simulink model "ADC_RoadRunner"  (R2024b)
settings: Solver=ode23tb  StartTime=0  StopTime=20  FixedStep=0.01  RelTol=1e-3
model workspace (MAT data in the model file):
  finalint = 0
  firstWarning = 1
  originalScenarioChecksum = '114339432DE22364D47BB28FC96DC10C'
undefined symbols (not defined in the file): curvature, DefaultGear, Defined, DEND_B, DEND_S, DEND_T, direction, DiscIntNeverNeededParam, driving, dspblkCoreblockFVToolHelper, Ego, fractalcoef, gcbh, gradbp, L, Lane, LF, LR, m, MAX_BRAKE, MAX_STEER, MAX_TORQUE, maxNumActors, MCAR, MIN_BRAKE, MIN_STEER, MIN_TORQUE, n, NUMD_B, NUMD_S, NUMD_T, Pose, psi_o, R, RRdamp, sigbuilder_block, STEER_RATIO, Tdead, thetaRefs, TrackWidth, ts, Ts, User, Vdead, Velocity, WB, xRef2s, yRef2s
libraries: simulink x9, roadrunnerscenario x7, simulink_extras x4, drivingscenarioandsensors x3, sensorinslib x2, robotalgslib x1, mpcadaslib x1, drivingvehiclecontroller x1, slpidlib x1, sensorgpslib x1, mspsensorlib x1, LaneDetection x1
(part 4 of 4)

== matlab function ADC_RoadRunner/Subsystem1/MATLAB Function ==
  data: ttc output; dist output; left output; right output; LL_avail output; RL_avail output; tend2stay output; ego input; act input; LaneBounds input; RoadSpeed input; ego_vel output; stay output; LL_Change output; RL_Change output; y_lane output; LCinProgress input
function [ttc,dist,left,right,LL_avail,RL_avail,tend2stay,ego_vel,stay,LL_Change,RL_Change,y_lane] = fcn(ego,act,LaneBounds,RoadSpeed, LCinProgress)                       


%% Major tasks to look into

% Check the performance while transitioning into another lane 
% Lane change output when the ego on extreme lanes.
% Develop code to handle lane changes on road curvatures
% Integrate with the trajectory generation and check the perfomance
% Convert the code to ego vehicle coordinates


%%
%define some parameters
r_c = 20; %range considered to MIOs
t_min =  2;

num_actors = length(act.Actors);
%num_lanes = length(LaneBounds.LaneBoundaries)-1;


%% Using sensor data 
% TracksNum = Tracking.NumTracks;
% 
% 
% for t = 1:TracksNum
%     ObjectID(t) = Tracking.Tracks(t).ObjectClassID;
%     TrackPos(:,t) = Tracking.Tracks(t).State(1:2:5);
%     TrackVel(:,t) = Tracking.Tracks(t).State(2:2:6);

%% ego position and  velocity magnitude
ego_pos = ego.Position;
ego_vel = ego.Velocity(1);  % velocity

%ttc: (array) : agent.relative position / abs(relative velocity)
ttc = zeros(1,num_actors);
left = zeros(1,num_actors);
right = zeros(1,num_actors);

dist =  zeros(1,num_actors);
tend2stay=1;

%%
y_lane = zeros(1,length(LaneBounds.LaneBoundaries))

for l=1:length(y_lane)
    y_lane(l)=LaneBounds.LaneBoundaries(l).Coordinates(end,2)
end

%%
for i= 1:num_actors

    % Grab actor positions and velocities
    actor_pos = act.Actors(i).Position;   
    actor_vel = act.Actors(i).Velocity(1);  % x-component velocity

    %relative velocity of the agent
    rel_vel = actor_vel - ego_vel;


    %% Check if the actor is within a r_c range. If it is out of range, pass lane change as '1' automatically.

   dist(i) = norm([actor_pos(1) actor_pos(2)]-[ego_pos(1) ego_pos(2)]);
        
    if dist(i) > r_c
        left(i)=1;
        right(i)=1;
        continue
    end

    %% Check if the actor is in the same lane as that of ego

    % If the actor and ego are in the same lane, it is considered a lead/following vehicle in the same lane and by defualt, the lane change flag is 1.

    if (actor_pos(2)< (ego_pos(2)+0.5) && actor_pos(2) > (ego_pos(2)-0.5))
        if (rel_vel < 0 && ego_vel < (RoadSpeed+5) && actor_pos(1) > ego_pos(1) )
            left(i) =1;
            right(i)=1;
            tend2stay=0;        % we need to incorporate too slow condition even when the relative velocity is greater than 0.

        elseif (rel_vel < 0 && ego_vel < (RoadSpeed+5) && actor_pos(1) < ego_pos(1) )
            left(i) =1;
            right(i)=1;
            tend2stay=1;
        end

        continue
    end

    
    %% calculate ttc for the rest of the vehicles


    ttc(i) = (actor_pos(1)-ego_pos(1))/abs(rel_vel);

    % checking conditions for other surrounding actors

    % all actors on the left lane of the ego vehicle
%%
    if actor_pos(2)-ego_pos(2) > 0  

        if and(rel_vel>0, ttc(i) > t_min)  % target vehicles on the front of ego vehicle (any lane)
    
            left(i)=1; 
            right(i)=1;
    
        elseif (ttc(i)<0 && rel_vel<0 && abs(ttc(i)) > t_min)    % target vehicle on the back of ego vehicle (ttc<0) (any lane)
            left(i) =1;
            right(i)=1;
    
        else 
            left(i) =0;
            right(i)=1;
    
        end

    % all actors on the right lane of the ego vehicle

    elseif actor_pos(2)-ego_pos(2) < 0
         
        if and(rel_vel>0, ttc(i) > t_min)  % target vehicles on the front of ego vehicle (any lane)
    
            left(i)=1;
            right(i)=1;
    
        elseif (ttc(i)<0 && rel_vel<0 && abs(ttc(i)) > t_min)    % target vehicle on the back of ego vehicle (ttc<0) (any lane)
            left(i) =1;
            right(i)=1;
    
        else 
            left(i) =1;
            right(i)=0;
    
        end
    end
%%

end

%% check if the vehicle is in the extreme end lanes

    if ego_pos(2)<y_lane(1) && ego_pos(2)>y_lane(2)

        LL=0; RL=1;
    elseif ego_pos(2) > y_lane(end) && ego_pos(2) < y_lane(end-1)
        RL=0; LL=1;
    else 

        RL=1;LL=1;
    end

%%
LL_avail = all(left) %&& LL;

RL_avail = all(right) %&& RL               %&& ~lcLeft ; this can be decided later 


%% final commands

stay = tend2stay || ~(tend2stay || LL_avail || RL_avail);
LL_Change =  ~tend2stay && LL_avail ;

RL_Change =  ~tend2stay && RL_avail && ~LL_Change ;
LCFlag = ~stay;
if LCFlag && LCinProgress
    LCFlag = false;
    stay = ~LCFlag;
end

%% 






end

== matlab function ADC_RoadRunner/Environment & Data/MATLAB Function ==
  data: states input; stateDynamics output; inputCmd input
function stateDynamics  = StateEstimator(states, inputCmd)


    % Model Parameters:
    J = 4000; 
    yawPolarIzz = 2050; %
    vehicleMass = 2000;
    lFront = 1.3425;
    lRear = 1.3425;
    corneringStiffnessFront = 12e3*100; 
    corneringStiffnessRear = 12e3*100;

    % Inputs
    accel = inputCmd(1);
    steerDelta = inputCmd(2);

    % States
    x = states(1);
    y = states(2);
    vx = states(3);
    vy = states(4);
    w = states(5);
    psi = states(6);
    
    

    alphaFront = atan2(vy + lFront*w)/vx - steerDelta;
    alphaRear = (vy - lRear*w)/vx;

    % Model - Dynamics Equations:
    stateDynamics = zeros(6,1);
    xDot = vx*cos(psi) - vy*sin(psi);
    yDot = vx*sin(psi)) + vy*cos(psi);

    vxDot = vy*w + 1/m();
    vyDot = ;
    psiDot = w;
    wDot = ;

    stateDynamics = [xDot; yDot; vxDot; vyDot; psiDot; wDot];

end

== stateflow chart ADC_RoadRunner/Vehicle Dynamics/Vehicle Dynamics/Engineer Steer Brake Dynamics/GearSelection1 ==
  state Park
    CurrGear = 0;
  state Reverse
    CurrGear = -1;
  state drive
    CurrGear = 1;
  (default) -> (junction 12)
  (junction 12) -> Reverse [order 3] : [DefaultGear == -1]
  (junction 12) -> drive [order 2] : [DefaultGear == 1]
  (junction 12) -> Park [order 1] : [DefaultGear == 0]
  (junction 12) -> Park [order 4] : %fallback to park
  drive -> Park [order 2] : [gear_cmd == 0 && allowShift(vc,Tbrake)]
  Park -> Reverse [order 2] : [gear_cmd == -1 && allowShift(vc,Tbrake)]
  Park -> drive [order 1] : [gear_cmd == 1 && allowShift(vc,Tbrake)]
  Reverse -> Park [order 2] : [gear_cmd == 0 && allowShift(vc,Tbrake)]
  drive -> Reverse [order 1] : [gear_cmd == -1 && allowShift(vc,Tbrake)]
  Reverse -> drive [order 1] : [gear_cmd == 1 && allowShift(vc,Tbrake)]
  data: Tdead parameter; Vdead parameter; vel function_input; brakeT function_input; allow function_output; CurrGear output; Tbrake input; vc input; gear_cmd input; DefaultGear parameter
  function allow = allowShift(vel, brakeT):
    | function allow = allowShift(vel, brakeT)
    | allow = (abs(vel) <= Vdead) && (abs(brakeT)>Tdead);
    | end

== matlab function ADC_RoadRunner/Vehicle Dynamics/Vehicle Dynamics/Engineer Steer Brake Dynamics/Compute Net Torque ==
  data: gear input; Tnet output; Tengine input; Tbrake input; vc input
function Tnet  = net_torque(gear,Tengine,Tbrake,vc)

%  --set engine torque based on current gear selection

if (gear == 0)
    %  --vehicle is in PARK, so force engine torque to zero
    Tengine = 0;
end

Tnet = Tengine + Tbrake*tanh(5*vc);

end

== matlab function ADC_RoadRunner/Vehicle Dynamics/Vehicle Dynamics/Engineer Steer Brake Dynamics/gear selection state machine ==
  data: gear output; gear_cmd input; vc input; Tbrake input; Tdead input; Vdead input
function gear = gear_change_FSM(gear_cmd,vc,Tbrake,Tdead,Vdead)

persistent GEAR

%  The vehicle gear can take on one of the following enumerated values:
%  -1 = REVERSE
%   0 = PARK
%   1 = DRIVE

%  --initialize the local persistent variables

if isempty(GEAR)
    %  --default gear at startup is PARK
    %  Note:  Change this to 1 if you want car to initialize in DRIVE
    GEAR = 0;
end


%  --evaluate the gear change finite state machine

switch GEAR
    case 0  % vehicle is in PARK
        if (gear_cmd == 1)
            %  --check to see if we can shift to DRIVE
            if ((abs(vc) <= Vdead) && (abs(Tbrake) > Tdead))
                %  --shift to DRIVE
                GEAR = 1;
            end
            
        elseif (gear_cmd == 2)
            %  --check to see if we can shift to REVERSE
            if ((abs(vc) <= Vdead) && (abs(Tbrake) > Tdead))
                %  --shift to REVERSE
                GEAR = 2;
            end
        end
        
    case 1  % vehicle is in DRIVE
        if (gear_cmd == 0)
            %  --check to see if we can shift to PARK
            if ((abs(vc) <= Vdead) && (abs(Tbrake) > Tdead))
                %  --shift to PARK
                GEAR = 0;
            end
            
        elseif (gear_cmd == 2)
            %  --check to see if we can shift to REVERSE
            if ((abs(vc) <= Vdead) && (abs(Tbrake) > Tdead))
                %  --shift to REVERSE
                GEAR = 2;
            end
        end
        
    case -1  % vehicle is in REVERSE
        if (gear_cmd == 0)
            %  --check to see if we can shift to PARK
            if ((abs(vc) <= Vdead) && (abs(Tbrake) > Tdead))
                %  --shift to PARK
                GEAR = 0;
            end
            
        elseif (gear_cmd == 1)
            %  --check to see if we can shift to DRIVE
            if ((abs(vc) <= Vdead) && (abs(Tbrake) > Tdead))
                %  --shift to DRIVE
                GEAR = 1;
            end
        end
        
    otherwise  %  --should never be here
        if (vc > Vdead)
            %  --moving forward, so must be in DRIVE
            GEAR = 1;
        elseif (vc < -Vdead)
            %  --moving backward, so must be in REVERSE
            GEAR = 2;
        else
            %  --vehicle stoppped, so must be in PARK
            GEAR = 0;
        end

end


%  --output the current actual gear setting

gear = GEAR;

return

== matlab function ADC_RoadRunner/Behavioural Planner/MATLAB Function3 ==
  data: Dest input; D2D output; CurrentPose input
function D2D = fcn(Dest, CurrentPose)
%CurrentPose(2) = -CurrentPose(2);
%D2D = norm(Dest - CurrentPose(1:2)');
Dest = [Dest(2) Dest(1)]; 
CurrentPose = [CurrentPose(2) CurrentPose(1)];
D2D = norm(Dest - CurrentPose(1:2));
% D2D=sqrt((CurrentPose(1)-Dest(1,1))^2+(CurrentPose(2)-Dest(1,2))^2);
end

== stateflow chart ADC_RoadRunner/Behavioural Planner/Chart ==
  settings: updateMethod=DISCRETE  sampleTime=Ts
  state Stationary
    en,du:
    VelCmd = 0;
    CurrentVelCmd = VelCmd;
    Navi = 0;
    Trans = 0;
    StopSim = 0;
    Tgap = 1;
    HoldBrake = 1;
    Braking = 0;
    SpeedUp = 0;
  state Navigation
    state RailCrossing [commented out]
      state Stop [commented out]
        en:
        VelCmd = 0;
        Braking = 1;
        CurrentVelCmd = VelCmd;
      state Approaching [commented out]
        en:
        Braking = 1;
        Tgap = 0;
        Trans = 0;
      state Transition [commented out]
        en:
        Tgap = 1;
        Trans = 1;
        Braking = 0;
        VelCmd = SceneSpeed;
        CurrentVelCmd = VelCmd;
      state ExitScene [commented out]
        en:
        ExitFlag = 1;
      (default) -> Navigation.RailCrossing.Approaching [commented out]
      Navigation.RailCrossing.Approaching -> Navigation.RailCrossing.Stop [commented out] : [D2S <= 6 && (RRCross == 1 || ObjectDist <= TransDist)]
      Navigation.RailCrossing.Transition -> Navigation.RailCrossing.Approaching [commented out] : [ObjectDist <= TransDist]
      Navigation.RailCrossing.Approaching -> Navigation.RailCrossing.Transition [commented out] : [RRCross == 0 && ObjectDist > TransDist && D2S <= 6]
      Navigation.RailCrossing.Stop -> Navigation.RailCrossing.Transition [commented out] : [RRCross == 0 && ObjectDist > TransDist]
      Navigation.RailCrossing.Approaching -> Navigation.RailCrossing.ExitScene [commented out] : [SceneID ~= 10]
      Navigation.RailCrossing.Transition -> Navigation.RailCrossing.ExitScene [commented out] : [SceneID == 0]
    state RoundAbout
      state Approaching
        en:
        Braking = 1;
        Trans = 0;
        Tgap = 0;
      state Stop
        en:
        VelCmd = 0;
        Braking = 1;
        CurrentVelCmd = VelCmd;
      state ExitScene
        en:
        ExitFlag = 1;
      state Transition
        en:
        Tgap = 1;
        Trans = 1;
        Braking = 0;
        VelCmd = SceneSpeed;
        CurrentVelCmd = VelCmd;
      (default) -> Navigation.RoundAbout.Approaching
      Navigation.RoundAbout.Approaching -> Navigation.RoundAbout.Stop [order 1] : [D2S <= 6]
      Navigation.RoundAbout.Stop -> Navigation.RoundAbout.Transition : [Clear2Go == 1]
      Navigation.RoundAbout.Approaching -> Navigation.RoundAbout.ExitScene [order 2] : [SceneID ~= 9]
      Navigation.RoundAbout.Transition -> Navigation.RoundAbout.ExitScene : [SceneID == 0]
    state DestCheck
      en,du:
      % dest reached?
      (default) -> (junction 47)
      (junction 47) -> (junction 48) [order 1] : [D2D < 2]
      (junction 47) -> (junction 49) [order 2] : {DestReached = 0;}
      (junction 48) -> (junction 50) : {DestReached = 1;}
      (junction 50) -> (junction 49) : {StopSim = 1;}
      (junction 49) -> (junction 51)
    state TrafficLight [commented out]
      note: Yellow light duration is 1s
      state Stop [commented out]
        en:
        Braking = 1;
        VelCmd = 0;
        CurrentVelCmd = VelCmd;
      state Approaching [commented out]
        en:
        Tgap = 0;
        Trans = 0;
        T2S = 0;
        %if TLstate(1,4) == 1
        Braking = 1;
        %else
        % ACC = 0;
        %end
      state DecisionOnYellow [commented out]
        en:
        T2S = D2S/EgoSpeed;
      state Transition [commented out]
        en:
        Trans = 1;
        Braking = 0;
        Tgap = 1;
        VelCmd = SceneSpeed;
        CurrentVelCmd = VelCmd;
      state ExitScene [commented out]
        en:
        ExitFlag = 1;
      DecisionOnYellow -> Navigation.TrafficLight.Approaching [commented out] : [T2S > 1.2]
      (default) -> Navigation.TrafficLight.Approaching [commented out]
      Navigation.TrafficLight.Approaching -> Navigation.TrafficLight.Stop [commented out] : [D2S <= 6]
      Navigation.TrafficLight.Stop -> Navigation.TrafficLight.Transition [commented out] : [TLstate(1,4) == 3 && ObjectDist > TransDist]
      Navigation.TrafficLight.Transition -> Navigation.TrafficLight.Approaching [commented out] : [TLstate(1,4) == 1  || ObjectDist < TransDist]
      Navigation.TrafficLight.Approaching -> Navigation.TrafficLight.Transition [commented out] : [TLstate(1,4) == 3 && ObjectDist > TransDist]
      Navigation.TrafficLight.Approaching -> Navigation.TrafficLight.ExitScene [commented out] : [SceneID ~= 8]
      Navigation.TrafficLight.Transition -> DecisionOnYellow [commented out] : [TLstate(1,4) == 2]
      DecisionOnYellow -> Navigation.TrafficLight.Transition [commented out] : [T2S <= 1.2]
      Navigation.TrafficLight.Transition -> Navigation.TrafficLight.ExitScene [commented out] : [SceneID == 0]
    state Drive
      en :
      HoldBrake = 0;
      SpeedUp = 1;
      VelCmd = RoadSpeed;
      CurrentVelCmd = VelCmd;
      ExitFlag = 0;
    state Go
      en:
      %VelCmd = RoadSpeed;
      %CurrentVelCmd = VelCmd;
      Trans = 0;
      ExitFlag = 0;
      Braking = 0;
      HoldBrake = 0;
      SpeedUp = 0;
    state StopSign
      state StoptSign4way
        state CheckInt
          du:
          % stopped?
          % ss priority?
        state CheckSS
          % stopped?
          % ss priority?
        state Transition
          en:
          % stay here while trans?!
          % while ~crossedLimitLine of TargetLane
          Trans = 1;
          Braking = 0;
          Tgap = 1;
          VelCmd = SceneSpeed;
          CurrentVelCmd = VelCmd;
        state ExitScene
          en:
          ExitFlag = 1;
        (default) -> Navigation.StopSign.StoptSign4way.CheckSS
        Navigation.StopSign.StoptSign4way.CheckSS -> Navigation.StopSign.StoptSign4way.CheckInt : [EgoSpeed < VelStop]
        Navigation.StopSign.StoptSign4way.CheckInt -> Navigation.StopSign.StoptSign4way.Transition : [egoSSPriority == 1 && Clear2Go == 1]
        Navigation.StopSign.StoptSign4way.Transition -> Navigation.StopSign.StoptSign4way.ExitScene : [SceneID == 0 && after(2,sec)]
      state SStype
        state Stop
          en:
          %VelCmd = 0;
          Braking = 1;
          SpeedUp = 0;
          CurrentVelCmd = VelCmd;
        state Approaching
          en:
          %VelCmd = ApproachingSpeed;
          % Braking = 1;
          Trans = 0;
          Tgap = 0;
        Navigation.StopSign.SStype.Stop -> 410 [order 1] : [numSS == 4]
        (default) -> Navigation.StopSign.SStype.Approaching
        Navigation.StopSign.SStype.Approaching -> Navigation.StopSign.SStype.Stop : [D2S <= 25]
        Navigation.StopSign.SStype.Stop -> 414 [order 2] : [numSS == 2]
      state StopSign2way
        state CheckInt
          en:
          %VelCmd = 0;
          HoldBrake = 1;
          CurrentVelCmd = VelCmd;
        state CheckSS
          % stopped?
          % ss priority?
        state Transition1
          en:
          % stay here while trans?!
          % while ~crossedLimitLine of TargetLane
          Trans = 1;
          Braking = 0;
          HoldBrake = 0;
          SpeedUp = 1;
          Tgap = 1;
          VelCmd = SceneSpeed;
          CurrentVelCmd = VelCmd;
        state ExitScene1
          en:
          ExitFlag = 1;
        (default) -> Navigation.StopSign.StopSign2way.CheckSS
        Navigation.StopSign.StopSign2way.CheckSS -> Navigation.StopSign.StopSign2way.CheckInt : [EgoSpeed < VelStop]
        Navigation.StopSign.StopSign2way.CheckInt -> Transition1 : [egoSSPriority == 1 && after(3,sec) && ToAClearance == 1]
        Transition1 -> Navigation.StopSign.StopSign2way.CheckInt [order 2] : [ToAClearance == 0]
        Transition1 -> ExitScene1 [order 1] : [SceneID == 0 && after(3,sec) && egoExit == 1]
      (default) -> SStype
      416 -> StoptSign4way
      411 -> StopSign2way
    Go -> RailCrossing [commented out] : [SceneID == 10]
    Drive -> RailCrossing [commented out] : [SceneID == 10]
    RailCrossing -> Go [commented out] : [ExitFlag == 1]
    Go -> RoundAbout [order 2] : [SceneID == 9]
    Drive -> RoundAbout [order 1] : [SceneID == 9]
    RoundAbout -> Go : [ExitFlag == 1]
    (default) -> DestCheck
    Drive -> TrafficLight [commented out] : [SceneID == 8]
    DestCheck -> Drive : [DestReached == 0]
    Go -> TrafficLight [commented out] : [SceneID == 8]
    Drive -> DestCheck [order 3] : [D2D < 2]
    TrafficLight -> Go [commented out] : [ExitFlag == 1]
    Drive -> StopSign [order 2] : [SceneID == 7]
    StopSign -> Go : [ExitFlag == 1]
    Go -> DestCheck [order 1] : [SceneID == 0]
    Go -> StopSign [order 3] : [SceneID == 7]
  (default) -> Stationary
  Stationary -> Navigation : [Navigate == 1]
  Navigation -> Stationary : [Navigate == 0 || DestReached == 1]
  data: TLstate input; numSS input; egoExit input; ToAClearance input; TransDist input; ApproachingSpeed input; EgoSpeed input; ObjectDist input; SceneSpeed input; SDist input; RRCross input; D2S input; DestReached local; Navigate input; ExitFlag local; D2D input; Clear2Go input; RoadSpeed input; CurrentVelCmd local; Navi local; VelCmd output; HoldBrake output; SceneID input; Tgap output; Trans output; StopSim output; Braking output; T2S local; VelStop input; egoSSPriority input; SpeedUp output

== matlab function ADC_RoadRunner/Behavioural Planner/MATLAB Function ==
  data: u input; y output
function y = fcn(u)

y = u;

== matlab function ADC_RoadRunner/Subsystem1/Subsystem/Function-Call Subsystem/MATLAB Function1 ==
  data: EgoPosition input; MIOPos input; curvature input; MIOVel input; V_i input; xd output; yd output; laneL input; laneR input; V_desired input; LCinProgress output
function [xd,yd,LCinProgress] = traj(EgoPosition,MIOPos,curvature,MIOVel, V_i, laneL, laneR, V_desired)
Vx_i =0;Vx_f=0;Vy_i=0;Vy_f=0;Ax_i=0;Ax_f=0;Ay_i=0;Ay_f=0;T_i=0;T_f=0;V_f=0;A_f=0;x_set=0;y_set=0;theta4=0;

P = zeros(6,6);
% xq = zeros(1,size(RefPath,1)); yq = zeros(1,size(RefPath,2));
EgoPosition(1,2)=-EgoPosition(1,2);
x_init= EgoPosition(1,1)+2; y_init = EgoPosition(1,2)-2;
% xq = RefPath(:,1)'; 
% yq = RefPath(:,2)';
num_foc_t = 98;
V_max= V_desired; ad_n=0; vd_n=MIOVel; wd_n=vd_n*curvature;
lane_width = 3.6 * (laneL-laneR); % +1 if left of current lane and -1 if right of current lane(rahul flipped)
xd = zeros(num_foc_t+1,1); 
yd = zeros(num_foc_t+1,1);
xf =0; 
yf = 0;

    %xf = [EgoPosition(1,1)+ MIOPos(1) ]; yf = [ EgoPosition(1,2)+ MIOPos(2) + lane_width];  
    xf = [EgoPosition(1,1)+ 20 ]; yf = [EgoPosition(1,2)+ lane_width]; % 80
    V_f = V_max;
    W_f = V_f*curvature;
    A_f = 0;

    %dist2crash = sqrt((x_init-MIOPos(1))^2+(y_init-MIOPos(2))^2);
    %dist2crash = 40;
    %T_f = abs(dist2crash/(MIOVel-V_i));
    T_f = 3;
    P = [1, T_i, T_i^2, T_i^3, T_i^4, T_i^5;
         0, 1, 2*T_i, 3*T_i^2, 4*T_i^3, 5*T_i^4;
         0, 0, 2, 6*T_i, 12*T_i^2, 20*T_i^3;
         1, T_f, T_f^2, T_f^3, T_f^4, T_f^5;
         0, 1, 2*T_f, 3*T_f^2, 4*T_f^3, 5*T_f^4;
         0, 0, 2, 6*T_f, 12*T_f^2, 20*T_f^3];

%     mtang4 = (yq(1,index+2)-yq(1,index+1))/(xq(1,index+2)-xq(1,index+1));

    Vx_i = vd_n*cos(theta4); 
    Vy_i = vd_n*sin(theta4); 
    Ax_i = ad_n*cos(theta4)-vd_n*sin(theta4)*wd_n; 
    Ay_i = ad_n*sin(theta4)+vd_n*cos(theta4)*wd_n;

%     if(xq(index+2)-xq(index+1)<0)
%         theta_4 = pi + atan(mtang4);
%     else
%         theta_4 = atan(mtang4);
%     end

    theta_4 =0;
    Vx_f = V_f*cos(theta_4); % curvature angle
    Vy_f = V_f*sin(theta_4);
    Ax_f = A_f*cos(theta_4)-V_f*sin(theta_4)*W_f;
    Ay_f = A_f*sin(theta_4)+V_f*cos(theta_4)*W_f;

    g1 = [x_init; Vx_i; Ax_i; xf; Vx_f; Ax_f];
    g2 = [y_init; Vy_i; Ay_i; yf; Vy_f; Ay_f];

    a_coeff = P\g1;
    b_coeff = P\g2;
    
    td = T_i;
    scatter(x_init,y_init,'go')
    hold on; 
    scatter(xf,yf,'ro')
    hold on;
    
    for f = 1:(num_foc_t+1)
        xd(f,1) = [1,td,td^2,td^3,td^4,td^5]*a_coeff 
        yd(f,1) = [1,td,td^2,td^3,td^4,td^5]*b_coeff
        td = td + (T_f - T_i)/num_foc_t;
        scatter(xd(f,1),yd(f,1),'y.');
    end

LCinProgress = 1;

% hold on;
end

== matlab function ADC_RoadRunner/Behavioural Planner/StopSignPriority ==
  settings: updateMethod=DISCRETE
  data: ToAClearance output; SDist input; D2S input; ObjTracks input; egoSSPriority output; SceneTracks input; egoPose input; egoSpeed input; numSS output; VelStop input; WB input; d output; flag input; flag output; midpoint input; midpoint output; egoExit output; egoEnter input; egoEnter output
function [ToAClearance, egoSSPriority, numSS, d, flag, midpoint, egoExit, egoEnter]  = StopSignPriority(SDist, D2S, ObjTracks, SceneTracks, egoPose, egoSpeed, VelStop, WB, flag, midpoint, egoEnter)
% calculate covariance matrix outside, input to this block is modified with final, unique detections

egoPose(2) = -egoPose(2);
egoPose(3) = -egoPose(3);
persistent SSPriority C1x C2y C3x C4y
% find stop signs + one of 2way or 4way or T-junction

% find number of signs (until we reach 0 valued columns)
numSS = 1;
for j = 1:length(SceneTracks(1,:))
    if any(SceneTracks(:,j))
        numSS = numSS + 1;
    end
end

% find number of cars
numCars = 0;
for j = 1:length(ObjTracks(1,:))
    if any(ObjTracks(:,j))
        numCars = numCars + 1;
    end
end


egoSSPriority = 1;
ToAClearance = 1;
% tempPriority = zeros(numCars+1,1);
d = zeros(10, 5); % distance, velocity, time, location (wrt ego), exit (leaving ints)
Objang = zeros(10, 1);
% priorityTable = zeros(numCars+1, 5);
egoExitang = egoPose(3) - atan2d(midpoint(2)-egoPose(2),midpoint(1)-egoPose(1)); % 0 deg = straight , + = right
egoExitdist = sqrt((midpoint(2)-egoPose(2))^2+(midpoint(1)-egoPose(1))^2);

if abs(egoExitang) >= 135 && egoExitdist >= 1 && egoEnter == 1
    d(1,5) = 1; % left the ints
    egoEnter = 0;
    flag = 0;
elseif abs(egoExitang) >= 135 && egoExitdist <= 10
    d(1,5) = 1;
end
egoExit = d(1,5) + 1;


% if D2S <= SDist || egoEnter == 1
% 
%     % [~, index] = min(abs(SceneTracks(1,:)'));
%     if numSS > 0
% 
%         Vmd = [-egoSpeed*sind(egoPose(3)), egoSpeed*cosd(egoPose(3))];
%         rot = [cosd(egoPose(3)) -sind(egoPose(3)); sind(egoPose(3)) cosd(egoPose(3))];
% 
%         % intersection region
%         if flag == 0
%             C1x = min(SceneTracks(1, 1:numSS)) - (WB + 3);
%             C2y = min(SceneTracks(3, 1:numSS)) - (WB + 3);
%             C3x = max(SceneTracks(1, 1:numSS)) + (WB + 3);
%             C4y = max(SceneTracks(3, 1:numSS)) + (WB + 3);
%             C1 = rot*[C1x; C2y] + egoPose(1:2)';
%             C2 = rot*[C3x; C4y] + egoPose(1:2)';
%             midpoint = (C1+C2)./2;
%             % midpoint = [2*egoPose(1)-C4y-C2y; 2*egoPose(2)+C1x+C3x]./2;
%         %   scatter(-SceneTracks(3,:)+egoPose(1),SceneTracks(1,:)+egoPose(2),'blue','filled')   
%             scatter(midpoint(1), midpoint(2), 'blue', 'filled')
%             rectangle('Position',[egoPose(1)-C4y egoPose(2)+C1x abs(C4y-C2y) abs(C3x-C1x)])
%             flag = C1x;
%         end
% 
% 
%         midpoint_ego = rot'*(midpoint - egoPose(1:2)');
%         % loop through num of cars (j)
% 
%         d(1,1) = sqrt((midpoint(1) - egoPose(1))^2 + (midpoint(2) - egoPose(2))^2);
%         d(1,2) = egoSpeed;
%         d(1,3) = d(1,1)/d(1,2);     %add ego TOA
%         d(1,4) = 4; % 4 is the location of the ego vehicle itself
% 
%         if d(1,1) <= 3
%             ToAThreshold = 1;
%         else
%             ToAThreshold = 3;
%         end
% 
%         if d(1,1) <= flag
%             egoEnter = 1;
%         end
% 
% 
%         % loop through signs (vectorized)
%         % if smallest dist 
%         % d(:,3) -> TOA = v/dist
% 
%         if numCars > 0
%             for k = 1:numCars
%                 d(k+1,1) = sqrt((midpoint_ego(2)-ObjTracks(3,k))^2+(midpoint_ego(1)-ObjTracks(1,k))^2); %sqrt((midpoint(1) - (-ObjTracks(3,k)+egoPose(1)))^2 + (midpoint(2) - (ObjTracks(1,k)+egoPose(2)))^2); 
%                 d(k+1,2) = sqrt((Vmd(1) - ObjTracks(2,k))^2 + (Vmd(2) - ObjTracks(4,k))^2);
%                 d(k+1,3) = d(k+1,1)/d(k+1,2); % TOA of other cars
%                 Objang(k) = atan2d(ObjTracks(1,k), -ObjTracks(3,k));
% 
%                 % Identify cars location (direction) wrt ego
%                 if Objang(k) <= 60
%                     d(k+1,4) = 1; % 1 = E, 2 = N, 3 = W
%                 elseif Objang(k) > 60  && Objang(k) < 120
%                     d(k+1,4) = 2; % 1 = E, 2 = N, 3 = W
%                 elseif Objang(k) >= 120
%                     d(k+1,4) = 3; % 1 = E, 2 = N, 3 = W
%                 end
% 
%                 % Identifying leaving cars
% 
%                 ActorHeading = atan2d(ObjTracks(2,k) - Vmd(1), -ObjTracks(4,k) - Vmd(2));
%                 actorExitang = ActorHeading - atan2d(midpoint_ego(1)-ObjTracks(1,k),midpoint_ego(2)+ObjTracks(3,k)); % 0 deg = straight , + = right
%                 %actorExitdist = sqrt((midpoint_ego(2)-ObjTracks(3,k))^2+(midpoint_ego(1)-ObjTracks(1,k))^2);
% 
% 
%                 if abs(actorExitang) >= 135 && d(k+1,1) >= 10 
%                     d(k+1,5) = 1; % left the ints
%                 else
%                     d(k+1,5) = 0; % did not leave
%                 end
% 
% 
%             end
% 
%             if numSS == 4 
%                 % Assign priorities based on rank TOA #1, before vehicle stops
%                 % d1 = d(d(:,1)~=0,:);
%                 [car, SSPriority] = sort(d(d(:,1)~=0 & d(:,5)==0));
%                 % priorityTable(:, 1:2) = [car, priority];
% 
%                 tempPriority = find(SSPriority == 1); % ego SS priority
%                 % for idx = 1:nn(vv<vv(find(nn==1)))
%                 % 
%                 % end
% 
%                 egoSSPriority = tempPriority(1);
% 
%             elseif numSS == 2
%                 [car, SSPriority] = sort(d((d(:,4)==2 | d(:,4)==4) & d(:,5)==0));
%                 tempPriority = find(SSPriority == 1); % ego SS priority
%                 egoSSPriority = tempPriority(1);
%                 ToAClearance = double(all(d(d(:,1)~=0 & d(:,5)==0 & d(:,4)~=4,3) > ToAThreshold));
% 
%             elseif numSS == 1
%                 [car, SSPriority] = sort(d((d(:,4)==2 | d(:,4)==4) & d(:,5)==0));
%                 tempPriority = find(SSPriority == 1); % ego SS priority
%                 egoSSPriority = tempPriority(1);
%                 ToAClearance = double(all(d(d(:,1)~=0 & d(:,5)==0 & d(:,4)~=4,3) > ToAThreshold));
% 
%             end
% 
%         end
%     end
% 
% 
% 
% 
%     % if egoSpeed <= VelStop
%     %     if SSPriority ~= 1
%     %         % for all vehicles with higher priority
%     %         % provide indicator signals to identify conflicts
%     %         % check indicator signs/conflicts and update priority based on that
%     %         % code to define leavingScene for other vehicles:
%     %         % update priority table
%     % 
%     %     end
%     % end
% 
% 
% 
% 
% 
% % elseif egoExit == 0
% 
% 
% end

== matlab function ADC_RoadRunner/Behavioural Planner/MATLAB Function1 ==
  data: EgoLength input; TransDist output; IntDist input
function TransDist = IntersectionClearanceDist(EgoLength,IntDist)

TransDist = IntDist + EgoLength;

== matlab function ADC_RoadRunner/Subsystem1/Subsystem/Turns LC in prog off ==
  data: u input; y output
function y = fcn(u)

persistent counter;
persistent input_high;

if isempty(counter)
    counter = 0;
end

if isempty(input_high)
    input_high = false;
end

if u ~= 0
    input_high = true;
end

if input_high && counter < 100
    y = u;
    counter = counter + 1;
else
    y = 0;
end

== matlab function ADC_RoadRunner/Controllers/Longitudinal Controllers/Subsystem/Distance to Traffic Sign ==
  data: currentDistanceTravelled input; relativeDistanceToScene output; signLatPose input; signLongPose input; ego_vel input; cumulativeDistance input; CurrentPose input; RefXY input; sceneDistance output; sceneDistance input; signPose output
function [relativeDistanceToScene, sceneDistance,signPose] = fcn(currentDistanceTravelled, signLatPose, signLongPose, ego_vel, cumulativeDistance, CurrentPose, RefXY, sceneDistance)

signPose=[40 40];
if signLongPose ~= 0
    % X front side of car, Y right side of car

    thetaSS = atan2d(signLongPose, signLatPose);

    
    beta = thetaSS+CurrentPose(3) - 90;
    alphaVector = norm([signLongPose, signLatPose]);
    xSS = alphaVector*cosd(beta);
    ySS = alphaVector*sind(beta);
    signPose = [xSS + CurrentPose(1), ySS + CurrentPose(2)];
    % signPose = [xSS - CurrentPose(2), ySS + CurrentPose(1)]; % y is x , x is -y

    
    %%%
    % signPose = [RefXY(end,1) RefXY(end,2)];

    distance = zeros(length(RefXY),1);
    for j = 1:length(RefXY)
        distance(j) = norm(signPose(1:2) - RefXY(j,1:2));
    end
    
    [~, ind] = mink(distance,2);
    
    if ind(1) > ind(2)
        ind = [ind(2); ind(1)];
    end

    signPoseOnPath = [0 0];
    m = 0; mm = 0; b = 0; bb = 0;
    m = (RefXY(ind(1),2) - RefXY(ind(2),2))/(RefXY(ind(1),1) - RefXY(ind(2),1));
    if m == 1e6
        signPoseOnPath = [RefXY(ind(1),1) signPose(2)];
    elseif m == 1e-6
        signPoseOnPath = [signPose(1) RefXY(ind(1),2)];
    else
        b = RefXY(ind(1),2) - m*RefXY(ind(1),1);
        mm = -1/m;
        bb = signPose(2) - mm*signPose(1);
        signPoseOnPath(1:2) = [(b-bb)/(mm-m) m*((b-bb)/(mm-m))+b];     
    end


    sceneDistance = cumulativeDistance(ind(1)) + norm(RefXY(ind(1),1:2) - signPoseOnPath(1:2)); % Distance to scene/sign, local origin
    relativeDistanceToScene = sceneDistance - currentDistanceTravelled - (2.6850 + 1); % Longitudinal Distance from Ego Vehicle to Scene
    relativeDistanceToScene = signLongPose - (2.6850 + 1);
    %%%
else

    relativeDistanceToScene = sceneDistance - currentDistanceTravelled - (2.6850 + 1);
end

end

== matlab function ADC_RoadRunner/Controllers/Longitudinal Controllers/MATLAB Function ==
  data: x output; u input; y output
function [x, y] = Function(u)
y = 0; x = 0;
y = u(1,1);
x = u(3,1);

== matlab function ADC_RoadRunner/Environment & Data/ENU to NWD/2D RefWaypoints ==
  data: Trajectory_Waypoints output; Initial_Yaw output; trajectory input; Initial_Position output; Destination_Position output
function [Trajectory_Waypoints, Initial_Yaw, Initial_Position, Destination_Position] = WaypointsExtract(trajectory) % This function takes all the available waypoints and replaces ...
                                                                            % ... the zeros following the final waypoint (x, y) with the final waypoint (x, y) 'k' times.

Trajectory_Length = 140; % Customize size [140, or 200, or 500 (RoadRunner maximum)], based on number of non-zero reference waypoints
Trajectory_Waypoints = zeros(Trajectory_Length, 2);

lastIndex = 1;
for i = 2:length(trajectory) % 500 points
    if norm(trajectory(i, 1:2)) == 0 % if sqrt(x^2 + y^2) == 0
        lastIndex = i-1; % use until previous waypoint
        break
    end
end

for j = 1:lastIndex
    Trajectory_Waypoints(j, 1:2) = trajectory(j, 1:2);
end

for k = (lastIndex+1):Trajectory_Length
    Trajectory_Waypoints(k, 1:2) = Trajectory_Waypoints(lastIndex, 1:2);
end

% Initial Yaw Angle
Initial_Yaw = atan2(trajectory(2,2) - trajectory(1,2),trajectory(2,1) - trajectory(1,1));

Destination_Position = Trajectory_Waypoints(lastIndex, 1:2);
Initial_Position = Trajectory_Waypoints(1, 1:2);

end

== matlab function ADC_RoadRunner/Subsystem1/Subsystem/PathPlanner/MATLAB Function3 ==
  settings: updateMethod=DISCRETE
  data: out output; check output; Xref input; Yref input; xd input; yd input; LC input; current_pos input; d2f input; dcheck output
function [out,check,dcheck]  = PathPlanning(Xref, Yref, xd, yd, LC, current_pos, d2f)

persistent output_matrix
persistent lc_triggered

if isempty(lc_triggered)
lc_triggered = false;
end

%lc_triggered=0;
%if isempty(hold_output)
  %  hold_output = false;
%end


if isempty(output_matrix)
    output_matrix = [Xref(:), Yref(:)];
    out = [Xref(:), Yref(:)];
else
    out = output_matrix;
end

if LC && ~isempty(xd) && ~isempty(yd)
    output_matrix = [xd(:), yd(:)];
    lc_triggered=true;
       
end

check=lc_triggered;
dcheck=output_matrix;
%out=output_matrix;

if lc_triggered && d2f < 5 %&& ~isempty(output_matrix) %&& ~hold_output
    %Yout = Yref(:);
    if current_pos > 0
        Xout = Xref(:);
        Yout = Yref + 3.6;
    else
        Xout = Xref(:);
        Yout = Yref;
    end
    output_matrix = [Xout, Yout];
    out=output_matrix;
    lc_triggered=false;
    %hold_output = true;
end

out=output_matrix;




%if ~LC && ~isempty(output_matrix) && lc_triggered
    %hold_output = false;
    %lc_triggered=false;
%end

end

== stateflow chart ADC_RoadRunner/Behavioural Planner/Routing ==
  state InitialRoute
    en:
    NewRoute = 0;
  state Rerouting
    en:
    NewRoute = 1;
  (default) -> InitialRoute
  InitialRoute -> Rerouting : [ReRoute == 1]
  Rerouting -> InitialRoute : [ReRoute == 0]
  data: ReRoute input; NewRoute output

== matlab function ADC_RoadRunner/Environment & Data/Waypoint Slicing ==
  data: x output; waypoints input; y output
function [x, y] = fcn(waypoints)

x = waypoints(:, 1);
y = waypoints(:, 2);

== matlab function ADC_RoadRunner/Environment & Data/GNSS // IMU Integration/MATLAB Function2 ==
  data: u input; y output; v input
function y = orientationError(u,v)
%ORIENTATIONERROR Compute the quaternion distance in degrees

%   Copyright 2019 The MathWorks, Inc.   

y = rad2deg(dist(quaternion(u), quaternion(v)));

== matlab function ADC_RoadRunner/Environment & Data/Vision & Tracking/MATLAB Function ==
  data: u input; target_idx_all output; target_idx output; track_state output
function [target_idx_all, target_idx, track_state] = fcn(u)
    TracksNum = u.NumTracks;
    target_idx_all = zeros(20,1);
    % track_state = zeros(20, 1);
    for k = 1:TracksNum
        target_idx_all(k) = u.Tracks(k).ObjectAttributes.TargetIndex;
    end
    target_idx = u.Tracks(1).ObjectAttributes.TargetIndex;
    track_state = u.Tracks(1).State;
end

== matlab function ADC_RoadRunner/Environment & Data/Global Coordinates to Ego Coordinates Conversion ==
  data: ActorsIn input; EgoVeh input; EgoRefActors output Bus: BusWorldToVehicleActors
function EgoRefActors  = GlobaltoEgoRefConv(ActorsIn,EgoVeh)
%ActorsOut = Simulink.Bus;
ActorsOut = ActorsIn;
numActors = length(ActorsIn.Actors);
for k = 1:numActors
    actorOut = driving.scenario.targetsToEgo(ActorsIn.Actors(k),EgoVeh);
    ActorsOut.Actors(k).ActorID             = actorOut.ActorID;
    ActorsOut.Actors(k).Position            = actorOut.Position;
    ActorsOut.Actors(k).Velocity            = actorOut.Velocity;
    ActorsOut.Actors(k).Roll                = actorOut.Roll;
    ActorsOut.Actors(k).Pitch               = actorOut.Pitch;
    ActorsOut.Actors(k).Yaw                 = actorOut.Yaw;
    ActorsOut.Actors(k).AngularVelocity    = actorOut.AngularVelocity;
end
EgoRefActors = ActorsOut;
end

== matlab function ADC_RoadRunner/Controllers/Longitudinal Controllers/Velocity Profiler ==
  data: CurrTime input; SpeedUp input; distanceToScene input; referenceVelocity output; BrakingPhase output; slowDownFlag input; safeStopDistance input; CurrVel input; desiredVelocity input; flag input; a_coeff input; flag output; a_coeff output; X_f input; X_f output; startTime input; startTime output
function [referenceVelocity, BrakingPhase, flag, a_coeff, X_f, startTime] = VelocityProfiler(CurrTime, SpeedUp, distanceToScene, slowDownFlag, safeStopDistance, CurrVel, desiredVelocity, flag, a_coeff, X_f, startTime)

BrakingPhase = 0;
D2S = abs(distanceToScene);
xx1 = 5;
SlowVel = 1;
t_i = 0;
t_f = 5;
referenceVelocity = desiredVelocity;

if ~slowDownFlag && ~SpeedUp
    referenceVelocity = desiredVelocity;
    flag = 0;
elseif ~slowDownFlag && SpeedUp
    if flag == 0
        flag = 1;
        startTime = CurrTime;
        t = CurrTime - startTime;
        P = [1, t_i, t_i^2, t_i^3, t_i^4, t_i^5;
             0, 1, 2*t_i, 3*t_i^2, 4*t_i^3, 5*t_i^4;
             0, 0, 2, 6*t_i, 12*t_i^2, 20*t_i^3;
             1, t_f, t_f^2, t_f^3, t_f^4, t_f^5;
             0, 1, 2*t_f, 3*t_f^2, 4*t_f^3, 5*t_f^4;
             0, 0, 2, 6*t_f, 12*t_f^2, 20*t_f^3];
    
        % Initial Conditions
        Vx_i = CurrVel; 
        Ax_i = 0; 
        Jx_i = 0;
        Vx_f = desiredVelocity;
        Ax_f = 0; 
        Jx_f = 0;
        InitialCond = [Vx_i; Ax_i; Jx_i; Vx_f; Ax_f; Jx_f];
        a_coeff = P\InitialCond;
        referenceVelocity = max([1,t,t^2,t^3,t^4,t^5]*a_coeff, 0);
    else
        t = CurrTime - startTime;
        if t > t_f
            referenceVelocity = desiredVelocity;
        else
            referenceVelocity = max([1,t,t^2,t^3,t^4,t^5]*a_coeff, 0);
        end
    
    end
 
elseif slowDownFlag && flag == 1
    flag = 0;
    X_i = 0;
    X_f = D2S - xx1; % Initial D2S at the moment when flag is raised (velocity poly starts from zero)

    P = [1, X_i, X_i^2, X_i^3, X_i^4, X_i^5;
         0, 1, 2*X_i, 3*X_i^2, 4*X_i^3, 5*X_i^4;
         0, 0, 2, 6*X_i, 12*X_i^2, 20*X_i^3;
         1, X_f, X_f^2, X_f^3, X_f^4, X_f^5;
         0, 1, 2*X_f, 3*X_f^2, 4*X_f^3, 5*X_f^4;
         0, 0, 2, 6*X_f, 12*X_f^2, 20*X_f^3];

    % Initial Conditions
    Vx_i = CurrVel; 
    Ax_i = 0; 
    Vx_f = SlowVel;
    Ax_f = -0.5; 
    Jx_i = 0;
    Jx_f = 0;
    InitialCond = [Vx_i; Ax_i; Jx_i; Vx_f; Ax_f; Jx_f];
    a_coeff = P\InitialCond;
    distCovered  = abs(X_f - (D2S - xx1));
    referenceVelocity = max([1,distCovered,distCovered^2,distCovered^3,distCovered^4,distCovered^5]*a_coeff, 0);
elseif slowDownFlag && flag == 0
    distCovered  = abs(X_f - (D2S - xx1));
    if D2S <= safeStopDistance + 0.5
        referenceVelocity = 0;
        BrakingPhase = 3;
    elseif D2S <= xx1
        referenceVelocity = SlowVel;
        BrakingPhase = 2;
    else
        BrakingPhase = 1;
        referenceVelocity = max([1,distCovered,distCovered^2,distCovered^3,distCovered^4,distCovered^5]*a_coeff, 0);
    end

end

end

== matlab function ADC_RoadRunner/Controllers/Longitudinal Controllers/Subsystem/Velocity - Curvature ==
  data: desiredVelocity input; referenceVelocity output; curveMinThreshold input; curvature input
function referenceVelocity = velocityCurveCalculation(desiredVelocity,curveMinThreshold, curvature)

    if abs(curvature) >= 0 && abs(curvature) <= curveMinThreshold
        referenceVelocity = desiredVelocity;
    else
        r = 1/abs(curvature);
        referenceVelocity = min(desiredVelocity, sqrt(9.81*r*0.9*0.4));
    end

== matlab function ADC_RoadRunner/Controllers/Longitudinal Controllers/Subsystem/Curvature Calculation ==
  data: RefXY input; curvatureAhead output; SlowdownDistance input; minimumCurvatureThreshold input; cumulativeDistance output
function [curvatureAhead, cumulativeDistance] = CurvatureCalculation(RefXY, SlowdownDistance, minimumCurvatureThreshold)

% minimumCurvatureThreshold: curvature value above which it is considered
% straight, not curved path

DX = gradient(RefXY(:, 1));
D2X = gradient(DX);
DY = gradient(RefXY(:,2));
D2Y = gradient(DY);
curvature = (DX.*D2Y - DY.*D2X) ./(DX.^2+DY.^2).^(3/2);

% Calculate Distance Vector
distanceMatrix = squareform(pdist(RefXY));
distanceSteps = zeros(length(RefXY)-1,1);
for i = 2:length(RefXY)
    distanceSteps(i-1,1) = distanceMatrix(i,i-1);
end
totalDistance = sum(distanceSteps); % Total distance travelled along reference path
cumulativeDistance = cumsum([0; distanceSteps]); % Distance for each waypoint

% Curvature Ahead Calculation
st = 0;
en = 1;
j1 = 1;
CurveInfo = zeros(length(curvature),7); % [startX startY endX endY MaxCurve startidx endidx]

for j = 1:length(curvature)
    if abs(curvature(j)) >= minimumCurvatureThreshold
        if abs(curvature(j)) >= CurveInfo(j1,5)
            CurveInfo(j1,5) = abs(curvature(j));
        end
        if st == 0
            CurveInfo(j1,1:2) = [RefXY(j,1) RefXY(j,2)]; % Startpoint
            CurveInfo(j1,6) = j;
            st = 1;
            en = 0;
        end
    elseif (abs(curvature(j)) < minimumCurvatureThreshold) && (en == 0)
            CurveInfo(j1,3:4) = [RefXY(j,1) RefXY(j,2)]; % Endpoint
            CurveInfo(j1,7) = j;
            j1 = j1+1;
            st = 0;
            en = 1;
    end
    if (j == length(curvature)) && (en == 0)
           CurveInfo(j1,3:4) = [RefXY(j,1) RefXY(j,2)]; % Endpoint
            CurveInfo(j1,7) = j;
            j1 = j1+1;
            st = 0;
            en = 1;
    end
end

j2 = 1;
curvatureAhead = zeros(length(curvature),1);
if j1 > 1
    for j = 1:length(cumulativeDistance)
        if (cumulativeDistance(j) >= (cumulativeDistance(CurveInfo(j2, 6)) - SlowdownDistance)) && (cumulativeDistance(j) < cumulativeDistance(CurveInfo(j2,7)))
            curvatureAhead(j) = CurveInfo(j2,5);
        elseif (cumulativeDistance(j) >= cumulativeDistance(CurveInfo(j2,7))) && (j2 < j1-1)
            curvatureAhead(j) = CurveInfo(j2,5);
            j2 = j2+1;
        else
            curvatureAhead(j) = curvature(j);
        end
    end
end

== matlab function ADC_RoadRunner/Controllers/Longitudinal Controllers/Subsystem/Reference Pose Search ==
  data: RefXY input; currentPose input; referenceCurvature input; curvature output; cumulativeDistance input; currentDistanceTravelled output
function [curvature, currentDistanceTravelled] = referencePoseSearch(RefXY, currentPose, referenceCurvature, cumulativeDistance)

dist = zeros(length(RefXY),1);
for j = 1:length(RefXY)
    dist(j) = norm(currentPose(1:2) - RefXY(j,1:2));
end

[~, ind] = mink(dist,2);

if ind(1) > ind(2)
    ind = [ind(2); ind(1)];
end

curvature = referenceCurvature(ind(1));
currentDistanceTravelled = cumulativeDistance(ind(1)) + norm(RefXY(ind(1),1:2) - currentPose(1:2));


% referencePoses = zeros(1, 2);
% m = 0; mm = 0; b = 0; bb = 0;
% m = (RefXY(ind(1),2) - RefXY(ind(2),2))/(RefXY(ind(1),1) - RefXY(ind(2),1));
% if m == inf
%     referencePoses = [RefXY(ind(1),1) currentPose(2)];
% elseif m == 0
%     referencePoses = [currentPose(1) RefXY(ind(1),2)];
% else
%     b = RefXY(ind(1),2) - m*RefXY(ind(1),1);
%     mm = -1/m;
%     bb = currentPose(2) - mm*currentPose(1);
%     referencePoses(1:2) = [(b-bb)/(mm-m) m*((b-bb)/(mm-m)) + b];
% 
% end
% positionError = norm(referencePoses(1:2) - currentPose(1:2));
